simulink model "mmcs_s2f"  (R2021b)
settings: Solver=FixedStepDiscrete  StartTime=0.0  StopTime=5  FixedStep=T_HF_TASK  RelTol=1e-3  EnableMultiTasking=on
PostLoadFcn:
  | run('init.m')
values from neighbouring files (symbols this model uses):
  ALIGN_DURATION = 700.0    [mmcs_s2f_dd.sldd]
  ALIGN_FINAL_CURRENT = 3277.0    [mmcs_s2f_dd.sldd]
  ALIGN_FINAL_SPEED = 0.0    [mmcs_s2f_dd.sldd]
  ALIGN_INIT_CURRENT = 1638.0    [mmcs_s2f_dd.sldd]
  ALIGN_THETA = 2731.0    [mmcs_s2f_dd.sldd]
  AMPTOS16 = 3277.0    [mmcs_s2f_dd.sldd]
  DIVSQRT_3 = 18918.0    [mmcs_s2f_dd.sldd]
  ENC_PT_CTRL = 4.0    [mmcs_s2f_dd.sldd]
  ENC_PULSE_NUM = 4000    [mmcs_s2f_dd.sldd]
  ENC_ST_CTRL = 2.0    [mmcs_s2f_dd.sldd]
  IF_ACC_DURATION = 1500.0    [mmcs_s2f_dd.sldd]
  IF_FINAL_CURRENT = 3277.0    [mmcs_s2f_dd.sldd]
  IF_FINAL_CURRENT_LOL = -3277.0    [mmcs_s2f_dd.sldd]
  IF_FINAL_CURRENT_UPL = 3277.0    [mmcs_s2f_dd.sldd]
  IF_FINAL_SPEED = 600.0    [mmcs_s2f_dd.sldd]
  IF_FINAL_SPEED_LOL = -600.0    [mmcs_s2f_dd.sldd]
  IF_FINAL_SPEED_UPL = 600.0    [mmcs_s2f_dd.sldd]
  IF_INIT_CURRENT = 1638.0    [mmcs_s2f_dd.sldd]
  INT16_MAX = 32767.0    [mmcs_s2f_dd.sldd]
  INT16_MIN = -32768.0    [mmcs_s2f_dd.sldd]
  MOTOR_F = 7.0E-6    [mmcs_s2f_dd.sldd]
  MOTOR_J = 2.8E-6    [mmcs_s2f_dd.sldd]
  MOTOR_PN = 4    [mmcs_s2f_dd.sldd]
  MOTOR_PNF = 4.0    [mmcs_s2f_dd.sldd]
  MOTOR_TL = 0.001    [mmcs_s2f_dd.sldd]
  PI_KI_PLL : value not decoded    [mmcs_s2f_dd.sldd]
  PI_KI_POS : value not decoded    [mmcs_s2f_dd.sldd]
  PI_KI_SPD : value not decoded    [mmcs_s2f_dd.sldd]
  PI_KI_TQ : value not decoded    [mmcs_s2f_dd.sldd]
  PI_KP_PLL : value not decoded    [mmcs_s2f_dd.sldd]
  PI_KP_POS : value not decoded    [mmcs_s2f_dd.sldd]
  PI_KP_SPD : value not decoded    [mmcs_s2f_dd.sldd]
  PI_KP_TQ : value not decoded    [mmcs_s2f_dd.sldd]
  PWM_FREQUENCY = 10000.0    [mmcs_s2f_dd.sldd]
  PWM_PERIOD_CYCLES = 7200.0    [mmcs_s2f_dd.sldd]
  RAD2RPM_F_DEN = 1000.0    [mmcs_s2f_dd.sldd]
  RAD2RPM_F_NUM = 9549.0    [mmcs_s2f_dd.sldd]
  RADTOS16_F = 10430.378350470453    [mmcs_s2f_dd.sldd]
  RADTOS16_I = 10430.0    [mmcs_s2f_dd.sldd]
  REF_CURRENT_LOL = -11470.0    [mmcs_s2f_dd.sldd]
  REF_CURRENT_UPL = 11470.0    [mmcs_s2f_dd.sldd]
  STM_ALIGN = 4.0    [mmcs_s2f_dd.sldd]
  STM_IFRUN = 5.0    [mmcs_s2f_dd.sldd]
  STM_INIT = 1.0    [mmcs_s2f_dd.sldd]
  STM_PTRUN = 7.0    [mmcs_s2f_dd.sldd]
  STM_START = 12.0    [mmcs_s2f_dd.sldd]
  STM_STRUN = 6.0    [mmcs_s2f_dd.sldd]
  STM_SWITCH = 11.0    [mmcs_s2f_dd.sldd]
  STO_C1 = 588    [mmcs_s2f_dd.sldd]
  STO_C2 = -5703    [mmcs_s2f_dd.sldd]
  STO_C3 = 1554    [mmcs_s2f_dd.sldd]
  STO_C4 = 7484    [mmcs_s2f_dd.sldd]
  STO_C5 = 1831    [mmcs_s2f_dd.sldd]
  STO_EST_MAX = 134213632.0    [mmcs_s2f_dd.sldd]
  STO_EST_MIN = -134213632.0    [mmcs_s2f_dd.sldd]
  STO_F1 = 4096.0    [mmcs_s2f_dd.sldd]
  STO_F2 = 4096.0    [mmcs_s2f_dd.sldd]
  STO_ST_CTRL = 3.0    [mmcs_s2f_dd.sldd]
  STOMS = 1000.0    [mmcs_s2f_dd.sldd]
  T_HF_TASK = 0.0001    [mmcs_s2f_dd.sldd]
  T_MF_TASK = 0.002    [mmcs_s2f_dd.sldd]
  TORQ_CTRL = 0.0    [mmcs_s2f_dd.sldd]
  U32MAXdivPulseNumber = 1073741    [mmcs_s2f_dd.sldd]
  VBUS = 24.0    [mmcs_s2f_dd.sldd]
undefined symbols (not defined in the file or in its folder): DiscIntNeverNeededParam
libraries: simulink x22, slpidlib x5, mcbplantlib x1, autolibpmsmexterior x1
(part 5 of 5)

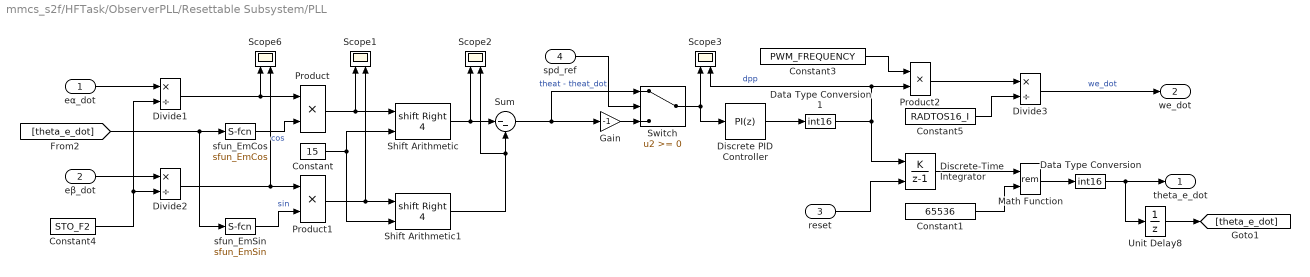
== system mmcs_s2f/HFTask/ObserverPLL/Resettable Subsystem/PLL ==
  eα_dot : Inport  OutDataTypeStr=int32
  eβ_dot : Inport  Port=2  OutDataTypeStr=int32
  reset : Inport  Port=3  OutDataTypeStr=uint8
  spd_ref : Inport  Port=4  OutDataTypeStr=int16
  Constant : Constant  Value=15  OutDataTypeStr=uint8
  Constant1 : Constant  Value=65536  OutDataTypeStr=int32
  Constant3 : Constant  Value=PWM_FREQUENCY  OutDataTypeStr=int32
  Constant4 : Constant  Value=STO_F2  OutDataTypeStr=int16
  Constant5 : Constant  Value=RADTOS16_I  OutDataTypeStr=uint16
  Data Type Conversion : DataTypeConversion  OutDataTypeStr=int16  RndMeth=Zero
  Data Type Conversion1 : DataTypeConversion  OutDataTypeStr=int16  RndMeth=Zero
  Discrete PID Controller : slpidlib/PID Controller  Controller=PI  Form=Parallel  TimeDomain=Discrete-time  UseExternalTs=off  SampleTime=-1  IntegratorMethod=Forward Euler  FilterMethod=Forward Euler  ControllerParametersSource=internal  P=PI_KP_PLL  I=PI_KI_PLL  D=0  UseFilter=on  N=100  TunerSelectOption=Transfer Function Based (PID Tuner App)  InitialConditionSource=internal  InitialConditionForIntegrator=0  InitialConditionForFilter=0  DifferentiatorICPrevScaledInput=0  ExternalReset=none  TrackingMode=off  Kt=1  LimitOutput=on  SatLimitsSource=internal  UpperSaturationLimit=1250  LowerSaturationLimit=-1250  LinearizeAsGain=off  AntiWindupMode=clamping  Kb=1  RndMeth=Zero  SaturateOnIntegerOverflow=on  PGainOutDataTypeStr=fixdt(1,32,16)  PProdOutDataTypeStr=fixdt(1,32,16)  POutMin=[]  POutMax=[]  IGainOutDataTypeStr=fixdt(1,32,16)  IProdOutDataTypeStr=fixdt(1,32,16)  IOutMin=[]  IOutMax=[]  DOutMin=[]  DOutMax=[]  NOutMin=[]  NOutMax=[]  SumOutDataTypeStr=int32  SumOutMin=[]  SumOutMax=[]  SaturationOutDataTypeStr=int32  SaturationOutMin=[]  SaturationOutMax=[]  PParamDataTypeStr=fixdt(1,32,16)  PParamMin=[]  PParamMax=[]  IParamDataTypeStr=fixdt(1,32,16)  IParamMin=[]  IParamMax=[]  DParamMin=[]  DParamMax=[]  NParamMin=[]  NParamMax=[]  KbParamMin=[]  KbParamMax=[]  KtParamMin=[]  KtParamMax=[]  KbOutMin=[]  KbOutMax=[]  KtOutMin=[]  KtOutMax=[]  IntegratorOutDataTypeStr=fixdt(1,32,16)  IntegratorOutMin=[]  IntegratorOutMax=[]  FilterOutMin=[]  FilterOutMax=[]  SumI1OutMin=[]  SumI1OutMax=[]  SumI2OutMin=[]  SumI2OutMax=[]  SumI3OutMin=[]  SumI3OutMax=[]  SumI4OutMin=[]  SumI4OutMax=[]  SumDOutMin=[]  SumDOutMax=[]  SumAccumDataTypeStr=fixdt(1,32,16)  DifferentiatorOutMin=[]  DifferentiatorOutMax=[]  FilterDiffOutCoefMin=[]  FilterDiffOutCoefMax=[]  ReciprocalOutMin=[]  ReciprocalOutMax=[]  SumDenOutMin=[]  SumDenOutMax=[]  SumNumOutMin=[]  SumNumOutMax=[]  DivideOutMin=[]  DivideOutMax=[]  UdiffTsProdOutMin=[]  UdiffTsProdOutMax=[]  NTsProdOutMin=[]  NTsProdOutMax=[]  UintegralTsProdOutMin=[]  UintegralTsProdOutMax=[]  UngainTsProdOutMin=[]  UngainTsProdOutMax=[]  IntegratorContinuousStateAttributes=''  IntegratorStateMustResolveToSignalObject=off  IntegratorRTWStateStorageClass=Auto  FilterContinuousStateAttributes=''  FilterStateMustResolveToSignalObject=off  FilterRTWStateStorageClass=Auto  ParallelPVariant=InternalParameters  IdealPVariant=Disabled  IVariant=InternalParameters  DVariant=Disabled  IntegratorVariant=Discrete  SatVariant=Enabled  AWVariant=DiscClampingParallel  PCopyVariant=Disabled  TRVariant=Disabled  FdbkBlocksVariant=Forward  IdealPFdbkVariant=Disabled  SatFdbkVariant=Disabled  DerivativeFilterVariant=Disabled  NVariant=Disabled  NCopyVariant=Disabled_SignalSpec  FilterICVariant=Disabled  IntegratorICVariant=InternalICs  ExternalResetVariant=Disabled  TRSumVariant=Passthrough  SumFdbkVariant=Disabled  SumVariant=Sum_PI  TsampFilterVariant=InternalTs  TsampNgainVariant=Passthrough  TsampIntegralVariant=Passthrough  ExternalSaturationOutDataTypeStr=Inherit: Same as second input
  Discrete-Time Integrator : DiscreteIntegrator  IntegratorMethod=Accumulation: Forward Euler  ExternalReset=rising  SampleTime=-1  OutDataTypeStr=int32  RndMeth=Zero  ICPrevOutput=DiscIntNeverNeededParam  ICPrevScaledInput=DiscIntNeverNeededParam
  Divide1 : Product  Inputs=*/  OutDataTypeStr=int16  RndMeth=Zero
  Divide2 : Product  Inputs=*/  OutDataTypeStr=int16  RndMeth=Zero
  Divide3 : Product  Inputs=*/  OutDataTypeStr=int16  RndMeth=Zero
  Gain : Gain  Gain=-1  OutDataTypeStr=int32  RndMeth=Zero
  Math Function : Math  Operator=rem  SaturateOnIntegerOverflow=on
  Product : Product  RndMeth=Zero
  Product1 : Product  RndMeth=Zero
  Product2 : Product  OutDataTypeStr=int32  RndMeth=Zero
  Scope{1..3,6} (4 alike) : Scope  NumInputPorts=2
  Shift Arithmetic : ArithShift  BitShiftNumberSource=Input port  BitShiftNumber=4  BitShiftDirection=Right
      settings: InputPortMap=u0,p1
  Shift Arithmetic1 : ArithShift  BitShiftNumberSource=Input port  BitShiftNumber=4  BitShiftDirection=Right
      settings: InputPortMap=u0,p1
  Sum : Sum  Inputs=|--  OutDataTypeStr=int32  RndMeth=Zero
  Switch : Switch  RndMeth=Zero
  Unit Delay8 : UnitDelay  SampleTime=-1  HasFrameUpgradeWarning=on
  sfun_EmCos : S-Function  FunctionName=sfun_EmCos  SFunctionDeploymentMode=off  EnableBusSupport=off  mask(Legacy Function){SFunctionSpec=int16 y1 = EmCos( int16 u1 ), ShowSpec=on}
      mask prompts: ShowSpec "显示函数设定"
      mask help:
      | 此模块允许您调用由以下代码继承工具定义指定的已有函数:
      | def.SFunctionName = 'sfun_EmCos';
      | def.OutputFcnSpec = 'int16 y1 = EmCos( int16 u1 )';
      | def.HeaderFiles = {'em_sincos.h'};
      | def.SourceFiles = {'em_sincos.c'};
      | def.IncPaths = {'.\c_code'};
      mask Help: <p>此模块是由代码继承工具自动生成的。有关此工具的详细帮助，请调用<a href="matlab:legacy_code('help')"> legacy_code('help')</a>.</p>
      mask Callback ShowSpec:
      | if strcmp(get_param(gcbh, 'ShowSpec'), 'on')
      |   set_param(gcbh, 'MaskDisplay', sprintf('fprintf(''%s'');', get_param(gcbh, 'SFunctionSpec')));
      | else
      |   set_param(gcbh, 'MaskDisplay', sprintf('fprintf(''%s'');', get_param(gcbh, 'FunctionName')));
      | end
      mask Display: fprintf('int16 y1 = EmCos( int16 u1 )');
  sfun_EmSin : S-Function  FunctionName=sfun_EmSin  SFunctionDeploymentMode=off  EnableBusSupport=off  mask(Legacy Function){SFunctionSpec=int16 y1 = EmSin( int16 u1 ), ShowSpec=on}
      mask prompts: ShowSpec "显示函数设定"
      mask help:
      | 此模块允许您调用由以下代码继承工具定义指定的已有函数:
      | def.SFunctionName = 'sfun_EmSin';
      | def.OutputFcnSpec = 'int16 y1 = EmSin( int16 u1 )';
      | def.HeaderFiles = {'em_sincos.h'};
      | def.SourceFiles = {'em_sincos.c'};
      | def.IncPaths = {'.\c_code'};
      mask Help: <p>此模块是由代码继承工具自动生成的。有关此工具的详细帮助，请调用<a href="matlab:legacy_code('help')"> legacy_code('help')</a>.</p>
      mask Callback ShowSpec:
      | if strcmp(get_param(gcbh, 'ShowSpec'), 'on')
      |   set_param(gcbh, 'MaskDisplay', sprintf('fprintf(''%s'');', get_param(gcbh, 'SFunctionSpec')));
      | else
      |   set_param(gcbh, 'MaskDisplay', sprintf('fprintf(''%s'');', get_param(gcbh, 'FunctionName')));
      | end
      mask Display: fprintf('int16 y1 = EmSin( int16 u1 )');
  theta_e_dot : Outport  OutDataTypeStr=int16
  we_dot : Outport  Port=2  OutDataTypeStr=int16
  wires:
  Product/1 -> Shift Arithmetic/1, Scope1/1
  Product1/1 -> Scope1/2, Shift Arithmetic1/1
  Constant/1 -> Shift Arithmetic1/2, Shift Arithmetic/2
  Shift Arithmetic/1 -> Sum/1, Scope2/1
  Shift Arithmetic1/1 -> Scope2/2, Sum/2
  reset/1 -> Discrete-Time Integrator/2
  Data Type Conversion/1 -> Unit Delay8/1, theta_e_dot/1
  Discrete-Time Integrator/1 -> Math Function/1
  Constant1/1 -> Math Function/2
  Math Function/1 -> Data Type Conversion/1
  Divide3/1 -> we_dot/1  "we_dot"
  [theta_e_dot] -> sfun_EmCos/1, sfun_EmSin/1
  sfun_EmSin/1 -> Product1/2  "sin"
  sfun_EmCos/1 -> Product/2  "cos"
  Sum/1 -> Switch/1, Gain/1  "theat - theat_dot"
  Divide1/1 -> Scope6/1, Product/1
  eα_dot/1 -> Divide1/1
  Constant4/1 -> Divide2/2, Divide1/2
  Divide2/1 -> Scope6/2, Product1/1
  eβ_dot/1 -> Divide2/1
  Constant3/1 -> Product2/1
  Product2/1 -> Divide3/1
  Constant5/1 -> Divide3/2
  Discrete PID Controller/1 -> Data Type Conversion1/1
  Data Type Conversion1/1 -> Discrete-Time Integrator/1, Scope3/2, Product2/2  "dpp"
  Unit Delay8/1 -> [theta_e_dot]
  Switch/1 -> Discrete PID Controller/1, Scope3/1
  Gain/1 -> Switch/3
  spd_ref/1 -> Switch/2

== system mmcs_s2f/MFTask/PosCtrlPlan/PosCtrlPlan/UpdatePosCtrl ==
  pos_ctrl : Inport  OutDataTypeStr=Bus: PosCtrlHandle_t
  Action Port : ActionPort  ActionPortLabel=if(u1 > 0)
  Data Store Write : DataStoreWrite  DataStoreName=pos_ctrl  DataStoreElements=pos_ctrl  IndexOptions=Index vector (dialog)  Indices=1  OutputSizes=1
  wires:
  pos_ctrl/1 -> Data Store Write/1

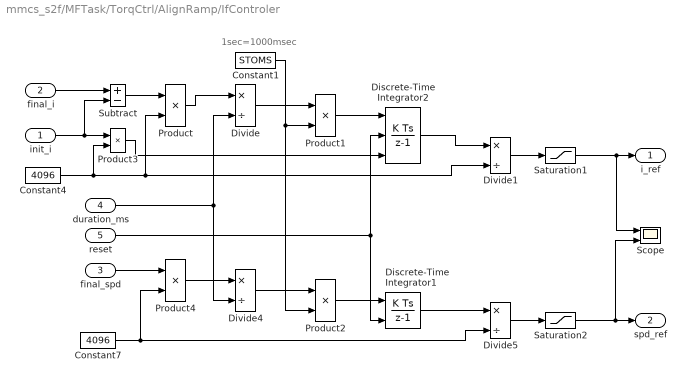
== system mmcs_s2f/MFTask/TorqCtrl/AlignRamp/IfControler ==
  note: 1sec=1000msec
  init_i : Inport  OutDataTypeStr=int16
  final_i : Inport  Port=2  OutDataTypeStr=int16
  final_spd : Inport  Port=3  OutDataTypeStr=int16
  duration_ms : Inport  Port=4  OutDataTypeStr=uint16
  reset : Inport  Port=5  OutDataTypeStr=uint8
  Constant1 : Constant  Value=STOMS  OutDataTypeStr=uint16
  Constant4 : Constant  Value=4096  OutDataTypeStr=uint16
  Constant7 : Constant  Value=4096  OutDataTypeStr=uint16
  Discrete-Time Integrator1 : DiscreteIntegrator  ExternalReset=level  SampleTime=-1  OutDataTypeStr=int32  RndMeth=Zero  ICPrevOutput=DiscIntNeverNeededParam  ICPrevScaledInput=DiscIntNeverNeededParam
  Discrete-Time Integrator2 : DiscreteIntegrator  ExternalReset=level  InitialConditionSource=external  SampleTime=-1  OutDataTypeStr=int32  RndMeth=Zero  ICPrevOutput=DiscIntNeverNeededParam  ICPrevScaledInput=DiscIntNeverNeededParam
  Divide{,1,4..5} (4 alike) : Product  Inputs=*/  OutDataTypeStr=int32  RndMeth=Zero
  Product{,1..4} (5 alike) : Product  OutDataTypeStr=int32  RndMeth=Zero
  Saturation1 : Saturate  UpperLimit=IF_FINAL_CURRENT_UPL  LowerLimit=IF_FINAL_CURRENT_LOL  OutDataTypeStr=int16  RndMeth=Zero
  Saturation2 : Saturate  UpperLimit=IF_FINAL_SPEED_UPL  LowerLimit=IF_FINAL_SPEED_LOL  OutDataTypeStr=int16  RndMeth=Zero
  Scope : Scope  NumInputPorts=2
  Subtract : Sum  Inputs=+-  OutDataTypeStr=int16  RndMeth=Zero
  i_ref : Outport
  spd_ref : Outport  Port=2  OutDataTypeStr=int16
  wires:
  Divide/1 -> Product1/1
  Saturation1/1 -> Scope/1, i_ref/1
  final_i/1 -> Subtract/1
  duration_ms/1 -> Divide/2, Divide4/2
  Product/1 -> Divide/1
  Divide1/1 -> Saturation1/1
  Discrete-Time Integrator2/1 -> Divide1/1
  Constant4/1 -> Product3/2, Product/2, Divide1/2
  Divide4/1 -> Product2/1
  final_spd/1 -> Product4/1
  Discrete-Time Integrator1/1 -> Divide5/1
  Divide5/1 -> Saturation2/1
  Constant7/1 -> Product4/2, Divide5/2
  Product4/1 -> Divide4/1
  Saturation2/1 -> Scope/2, spd_ref/1
  reset/1 -> Discrete-Time Integrator2/2, Discrete-Time Integrator1/2
  Product1/1 -> Discrete-Time Integrator2/1
  Product2/1 -> Discrete-Time Integrator1/1
  Constant1/1 -> Product1/2, Product2/2
  init_i/1 -> Subtract/2, Product3/1
  Product3/1 -> Discrete-Time Integrator2/3
  Subtract/1 -> Product/1

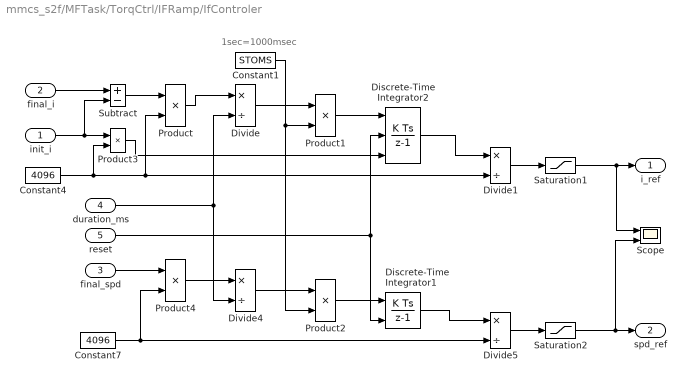
== system mmcs_s2f/MFTask/TorqCtrl/IFRamp/IfControler ==
  note: 1sec=1000msec
  init_i : Inport  OutDataTypeStr=int16
  final_i : Inport  Port=2  OutDataTypeStr=int16
  final_spd : Inport  Port=3  OutDataTypeStr=int16
  duration_ms : Inport  Port=4  OutDataTypeStr=uint16
  reset : Inport  Port=5  OutDataTypeStr=uint8
  Constant1 : Constant  Value=STOMS  OutDataTypeStr=uint16
  Constant4 : Constant  Value=4096  OutDataTypeStr=uint16
  Constant7 : Constant  Value=4096  OutDataTypeStr=uint16
  Discrete-Time Integrator1 : DiscreteIntegrator  ExternalReset=level  SampleTime=-1  OutDataTypeStr=int32  RndMeth=Zero  ICPrevOutput=DiscIntNeverNeededParam  ICPrevScaledInput=DiscIntNeverNeededParam
  Discrete-Time Integrator2 : DiscreteIntegrator  ExternalReset=level  InitialConditionSource=external  SampleTime=-1  OutDataTypeStr=int32  RndMeth=Zero  ICPrevOutput=DiscIntNeverNeededParam  ICPrevScaledInput=DiscIntNeverNeededParam
  Divide{,1,4..5} (4 alike) : Product  Inputs=*/  OutDataTypeStr=int32  RndMeth=Zero
  Product{,1..4} (5 alike) : Product  OutDataTypeStr=int32  RndMeth=Zero
  Saturation1 : Saturate  UpperLimit=IF_FINAL_CURRENT_UPL  LowerLimit=IF_FINAL_CURRENT_LOL  OutDataTypeStr=int16  RndMeth=Zero
  Saturation2 : Saturate  UpperLimit=IF_FINAL_SPEED_UPL  LowerLimit=IF_FINAL_SPEED_LOL  OutDataTypeStr=int16  RndMeth=Zero
  Scope : Scope  NumInputPorts=2
  Subtract : Sum  Inputs=+-  OutDataTypeStr=int16  RndMeth=Zero
  i_ref : Outport
  spd_ref : Outport  Port=2  OutDataTypeStr=int16
  wires:
  Divide/1 -> Product1/1
  Saturation1/1 -> Scope/1, i_ref/1
  final_i/1 -> Subtract/1
  duration_ms/1 -> Divide/2, Divide4/2
  Product/1 -> Divide/1
  Divide1/1 -> Saturation1/1
  Discrete-Time Integrator2/1 -> Divide1/1
  Constant4/1 -> Product3/2, Product/2, Divide1/2
  Divide4/1 -> Product2/1
  final_spd/1 -> Product4/1
  Discrete-Time Integrator1/1 -> Divide5/1
  Divide5/1 -> Saturation2/1
  Constant7/1 -> Product4/2, Divide5/2
  Product4/1 -> Divide4/1
  Saturation2/1 -> Scope/2, spd_ref/1
  reset/1 -> Discrete-Time Integrator2/2, Discrete-Time Integrator1/2
  Product1/1 -> Discrete-Time Integrator2/1
  Product2/1 -> Discrete-Time Integrator1/1
  Constant1/1 -> Product1/2, Product2/2
  init_i/1 -> Subtract/2, Product3/1
  Product3/1 -> Discrete-Time Integrator2/3
  Subtract/1 -> Product/1

== matlab function mmcs_s2f/AngleSinM2E/AngleAbs2Sin ==
  data: u input; y output
function y = fcn(u)
if (u > pi)
    y = u - 2*pi;
elseif (u < -pi)
    y = u + 2*pi;
else
    y = u;
end

== matlab function mmcs_s2f/SpeedConvert/SpdConvSto/GetAvgVal ==
  data: in_data input int16; avg output int16
function avg = GetAvgVal(in_data)
    persistent buff;
    persistent index;
    
    BUFF_SIZE = 16;
    
    % Initialize buffer and index on first call
    if isempty(buff)
        buff = zeros(1, BUFF_SIZE, 'int16');
        index = 1;
    end
    
    % Put new data in buffer
    buff(index) = in_data;
    index = index + 1;
    if index > BUFF_SIZE
        index = 1;
    end
    
    % Calculate buffer average value
    sum = int32(0);
    for i = 1:BUFF_SIZE
        sum = sum + int32(buff(i));
    end
    avg = int16(sum / BUFF_SIZE);
end

== stateflow chart mmcs_s2f/MFTask/Chart ==
  state PT_RUN
    stm_state = STM_PTRUN;
  state ST_RUN
    stm_state = STM_STRUN;
    ex:
    if(sys_ctrl_mode == STO_ST_CTRL)
    align_comp = 0;
    end
  state SWITCH
    stm_state = STM_SWITCH;
  state PREPARE
    stm_state = STM_PREPARE;
    en,du,ex:
    ct_ctrl_mode = TORQ_CTRL;
    if(sys_ctrl_mode == HALL_ST_CTRL)
    align_comp = 1;
    end
    if(align_comp == 1)
    if((sys_ctrl_mode == ENC_ST_CTRL) || ...
    (sys_ctrl_mode == HALL_ST_CTRL))
    ct_ctrl_mode = SPD_CTRL;
    elseif(sys_ctrl_mode == ENC_PT_CTRL)
    ct_ctrl_mode = POS_CTRL;
    end
    end
  state INIT
    stm_state = STM_INIT;
    ct_ctrl_mode = TORQ_CTRL;
  state START
    stm_state = STM_START;
  state IF_RUN
    stm_state = STM_IFRUN;
  state IDLE
    stm_state = STM_IDLE;
  state ANY_STOP
    stm_state = STM_ANY_STOP;
  state ALIGN
    stm_state = STM_ALIGN;
    ex:
    align_comp = 1;
  state STOP_IDLE
    stm_state = STM_STOP_IDLE;
  state STOP
    stm_state = STM_STOP;
  START -> PT_RUN [order 4] : [ct_ctrl_mode == POS_CTRL]
  PT_RUN -> ANY_STOP : [motor_start == 0]
  START -> ST_RUN [order 1] : [ct_ctrl_mode == SPD_CTRL]
  ST_RUN -> ANY_STOP : [motor_start == 0]
  SWITCH -> ST_RUN
  IF_RUN -> SWITCH [order 2] : [(sys_ctrl_mode == STO_ST_CTRL) && (after(IF_ACC_DURATION, msec)) && (transition)]{ct_ctrl_mode = SPD_CTRL;}
  (default) -> INIT
  IF_RUN -> ANY_STOP [order 1] : [motor_start == 0]
  PREPARE -> START : [after(2, msec)]
  IDLE -> PREPARE : [motor_start]
  START -> IF_RUN [order 3] : [align_comp && (ct_ctrl_mode == TORQ_CTRL)]
  INIT -> IDLE
  ALIGN -> ANY_STOP : [after(ALIGN_DURATION, msec)]
  ANY_STOP -> STOP
  STOP_IDLE -> IDLE : [after(100, msec)]
  START -> ALIGN [order 2] : [align_comp == 0]
  STOP -> STOP_IDLE : [after(100, msec)]
  data: stm_state output uint8 =uint8(1); motor_start input uint8; align_comp local =uint8(0); STM_PREPARE parameter; STM_ALIGN parameter; STM_IFRUN parameter; STM_STRUN parameter; STM_INIT parameter; STM_IDLE parameter; STM_STOP parameter; ct_ctrl_mode output; STM_PTRUN parameter; sys_ctrl_mode input; SPD_CTRL parameter; POS_CTRL parameter; ENC_ST_CTRL parameter; ENC_PT_CTRL parameter; TORQ_CTRL parameter; STM_ANY_STOP parameter; STM_STOP_IDLE parameter; transition input; STO_ST_CTRL parameter; STM_SWITCH parameter; ALIGN_DURATION parameter; STM_START parameter; IF_ACC_DURATION parameter; HALL_ST_CTRL parameter; IF_CTRL parameter; MOTOR_TYPE parameter; MOTOR_TYPE_TG5P60 parameter; MOTOR_TYPE_TB2P parameter; MOTOR_TYPE_JSF630 parameter
